simulink model "full_modek"  (R2024b)
settings: Solver=VariableStepAuto  StartTime=0.0  StopTime=20  RelTol=1e-3
values from neighbouring files (symbols this model uses):
  C = [1 0 0 0; 0 1 0 0]    [Car_test_UDP.m]    (also in Final_Code_GPS.m; Final_Code_plotting_reset_kalman.m; KalmanFilter.m)
undefined symbols (not defined in the file or in its folder): Sim3dSensor
libraries: sim3dautolib x4, sim3dcameralib x1, sim3dlib x1
settings Model: Creator=The MathWorks, Inc.  LastModifiedBy=ritvi
settings SolverCC: AlgebraicLoopSolver=TrustRegion
settings OptimizationCC: ReuseModelBlockBuffer=off
settings DebuggingCC: UnconnectedInputMsg=warning  UnconnectedOutputMsg=warning  UnconnectedLineMsg=warning  SymbolicDimsDataTypeCodeGenerationDiagnostic=none
settings ModelReferenceCC: EnableRefExpFcnMdlSchedulingChecks=on
settings RTWCC: GPUComputeCapability=3.5  DLArmComputeVersion=19.05

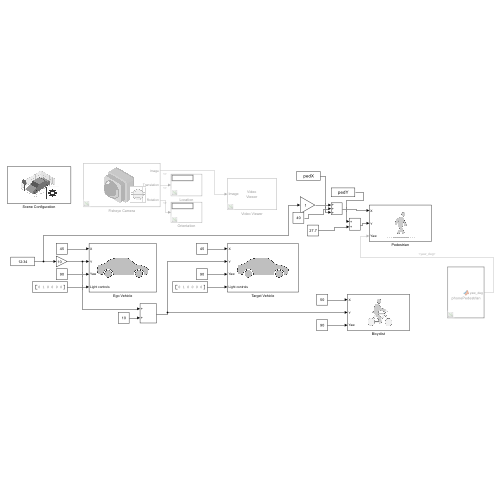
[thumbnail: Simulink's stored preview of the top-level diagram]
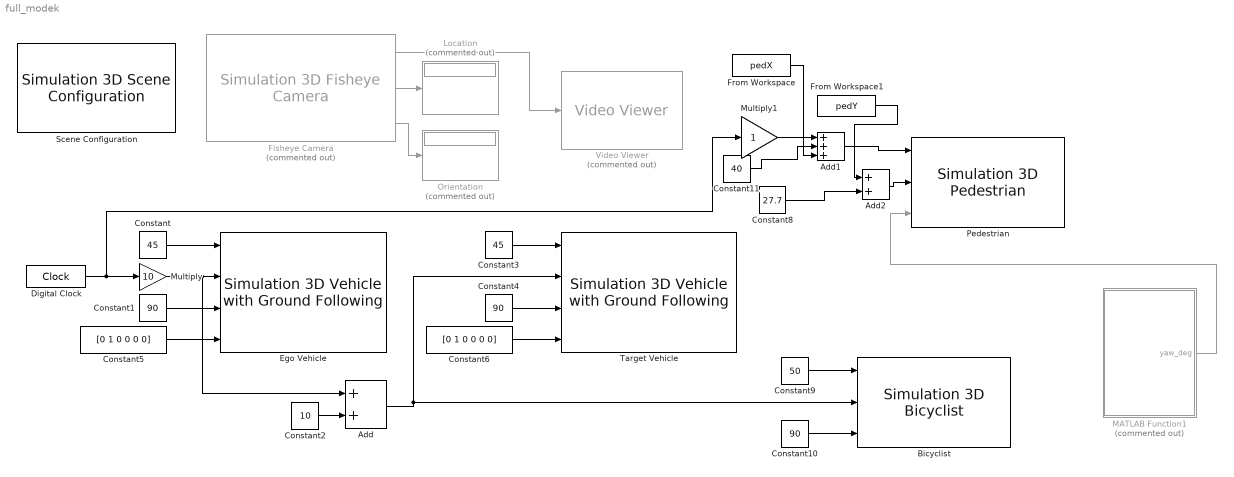
== system full_modek ==
  Add : Sum
  Add1 : Sum  Inputs=+++
  Add2 : Sum
  Bicyclist : sim3dautolib/Simulation 3D Bicyclist  Priority=-1  Scale=[1, 1, 1]  InitialPos=[0, 0, 0]  InitialRot=[0, 0, 0]  ActorName=SimulinkBicyclist1  SampleTime=-1  ActorType=SimulinkBicyclist  ActorTag=SimulinkBicyclist1  ID=1  aMode=3  CoordinateScheme=ISO  TransformOutportEnabled=off
      settings: LibrarySourceBlock=drivingsim3d/Simulation 3D Bicyclist
  Constant : Constant  Value=45
  Constant1 : Constant  Value=90
  Constant10 : Constant  Value=90
  Constant11 : Constant  Value=40
  Constant2 : Constant  Value=10
  Constant3 : Constant  Value=45
  Constant4 : Constant  Value=90
  Constant5 : Constant  Value=[0 1 0 0 0 0]
  Constant6 : Constant  Value=[0 1 0 0 0 0]
  Constant8 : Constant  Value=27.7
  Constant9 : Constant  Value=50
  Digital Clock : DigitalClock  SampleTime=0.01
  Ego Vehicle : sim3dautolib/Simulation 3D Vehicle with Ground Following  Priority=-1  PassVehMesh=Hatchback  MeshPath=/MathWorksSimulation/Vehicles/Muscle/Meshes/SK_MuscleCar.SK_MuscleCar  TrackWidth=1.9  WheelBase=3  WheelRadius=0.35  VehColor=Red  InitialPos=[45, 0, 0]  InitialRot=[0, 0, 90]  ActorName=EgoVehicle  SampleTime=-1  ActorType=SimulinkVehicle  ID=C  aMode=3  ActorTag=EgoVehicle  CoordinateScheme=ISO  VehLightsControl=on  HeadlightColor=[ 1, 1, 1 ]  HighBeamIntensity=100000  LowBeamIntensity=60000  HighBeamConeAngle=70  LowBeamConeAngle=70  LeftHeadlightOrientation=[ 0, 0 ]  RightHeadlightOrientation=[ 0, 0 ]  BrakelightIntensity=500  ReverselightIntensity=500  SignallightIntensity=500  SignallightPeriod=1  SignalPulseWidth=50  TransformOutportEnabled=off
      settings: LibrarySourceBlock=drivingsim3d/Simulation 3D Vehicle with Ground Following
  Fisheye Camera : sim3dcameralib/Simulation 3D Fisheye Camera  Priority=1  Commented=on  sensorTag=Sim3dSensor�  sensorId=1  sensorName=Sim3dSensor�  vehTagList={'EgoVehicle';'Scene Origin';'TargetVehicle'}  vehTag=EgoVehicle  mountLoc=Roof center  offsetFlag=off  tmountOffset=[0, 0, 0]  extTmount=off  rmountOffset=[0, 0, 0]  extRmount=off  OpticalCenter=[640, 360]  ImageSize=[720, 1280]  RadialDistortion=[320, -0.0005, 0, 0]  StretchMatrix=[1, 0; 0, 1]  TransformOutportEnabled=on  SampleTime=-1  mountPoint=[0 0 1.56]  mountOrientation=[0 0 0]  aMode=3  ID=1
      settings: LibrarySourceBlock=drivingsim3d/Simulation 3D Fisheye Camera
  From Workspace : FromWorkspace  VariableName=pedX
  From Workspace1 : FromWorkspace  VariableName=pedY
  Location : Display  Commented=on
  MATLAB Function1 : MATLAB Function  Commented=on  TreatAsAtomicUnit=on
  Multiply : Gain  Gain=10
  Multiply1 : Gain
  Orientation : Display  Commented=on
  Pedestrian : sim3dautolib/Simulation 3D Pedestrian  Priority=-1  PedestrianType=Female 1  Scale=[1, 1, 1]  InitialPos=[0, 0, 0]  InitialYaw=0  ActorName=SimulinkPedestrian1  SampleTime=-1  ActorType=SimulinkPedestrian  ActorTag=SimulinkPedestrian1  ID=1  aMode=3  CoordinateScheme=ISO  TransformOutportEnabled=off
      settings: LibrarySourceBlock=drivingsim3d/Simulation 3D Pedestrian
  Scene Configuration : sim3dlib/Simulation 3D Scene Configuration  Priority=0  ProjectFormat=Unreal Editor  SceneDesc=Large parking lot  ProjectName=C:\Program Files\MATLAB\R2024b\toolbox\shared\sim3d_projects\automotive_project_windows\UE\WindowsNoEditor\VehicleSimulation.exe  ScenePath=/Game/Maps/HwStrght  UEProjPath=C:\Local\AutoVrtlEnv\AutoVrtlEnv.uproject  EnableOpenDRIVE=off  vehTagList={'Custom';'EgoVehicle';'Scene Origin';'TargetVehicle'}  vehTag=EgoVehicle  FreeCameraInitialTranslation=[0, 0, 0]  FreeCameraDefaultInitialTranslation=[-6, 0, 2]  FreeCameraInitialRotation=[0, 0, 0]  FreeCameraDefaultInitialRotation=[0, -15, 0]  OpVisEn=off  Ts=1/60  EnableWindow=on  EnableRemoteAccess=off  EnableWeather=off  SunAzimuth=183.600  SunAltitude=0.0  EnableGeospatialSun=off  Latitude=0  Longitude=0  Date=2023-01-01  Time=10:30:00  GeoTimeZone=-5.0  SunDaylightSaving=off  wind=1  clouds=50.0  EnableVolumetricClouds=off  CloudCoverage=0  CloudAltitude=6  fog=0.0  rain=18.0  RaindropsEffect=off  SnowDensity=0  EnableGeospatial=off  UseTrueOrigin=off  OriginHeight=200  OriginLatitude=40.744652  OriginLongitude=-73.988864  MapStyle=Aerial  AdditionalAssetIDs=[]  UseAdvancedSunSky=off  SolarTime=11  TimeZone=-5  Day=21  Month=9  Year=2022  UseDaylightSavingTime=on  DSTStartDay=10  DSTStartMonth=3  DSTEndDay=3  DSTEndMonth=11  DSTSwitchHour=2  sensorTag=MainCamera2  sensorId=2  sensorName=MainCamera2  mountLoc=Origin  offsetFlag=off  tmountOffset=[0, 0, 0]  rmountOffset=[0, 0, 0]  HorizontalResolution=1280  VerticalResolution=720  HorizontalFOV=60  mountPoint=[0 0 0]  mountOrientation=[0 0 0]  aMode=3  ID=2  GeoTrigger=Inactive
      settings: LibrarySourceBlock=drivingsim3d/Simulation 3D Scene Configuration
  Target Vehicle : sim3dautolib/Simulation 3D Vehicle with Ground Following  Priority=-1  PassVehMesh=Sport utility vehicle  MeshPath=/MathWorksSimulation/Vehicles/Muscle/Meshes/SK_MuscleCar.SK_MuscleCar  TrackWidth=1.9  WheelBase=3  WheelRadius=0.35  VehColor=Green  InitialPos=[45, 10, 0]  InitialRot=[0, 0, 90]  ActorName=TargetVehicle  SampleTime=-1  ActorType=SimulinkVehicle  ID=C  aMode=3  ActorTag=TargetVehicle  CoordinateScheme=ISO  VehLightsControl=on  HeadlightColor=[ 1, 1, 1 ]  HighBeamIntensity=100000  LowBeamIntensity=60000  HighBeamConeAngle=70  LowBeamConeAngle=70  LeftHeadlightOrientation=[ 0, 0 ]  RightHeadlightOrientation=[ 0, 0 ]  BrakelightIntensity=500  ReverselightIntensity=500  SignallightIntensity=500  SignallightPeriod=1  SignalPulseWidth=50  TransformOutportEnabled=off
      settings: LibrarySourceBlock=drivingsim3d/Simulation 3D Vehicle with Ground Following
  Video Viewer : VideoViewer  Commented=on  FigPos=[993.8 1062.8 530.4 429.6]
  wires:
  Multiply/1 -> Add/1, Ego Vehicle/2
  Constant/1 -> Ego Vehicle/1
  Constant1/1 -> Ego Vehicle/3
  Constant2/1 -> Add/2
  Add/1 -> Target Vehicle/2, Bicyclist/2
  Fisheye Camera/1 -> Video Viewer/1
  Digital Clock/1 -> Multiply1/1, Multiply/1
  Fisheye Camera/2 -> Location/1
  Fisheye Camera/3 -> Orientation/1
  Constant3/1 -> Target Vehicle/1
  Constant4/1 -> Target Vehicle/3
  Constant5/1 -> Ego Vehicle/4
  Constant6/1 -> Target Vehicle/4
  MATLAB Function1/1(yaw_deg) -> Pedestrian/3
  Constant9/1 -> Bicyclist/1
  Constant10/1 -> Bicyclist/3
  Multiply1/1 -> Add1/1
  Add1/1 -> Pedestrian/1
  Constant11/1 -> Add1/2
  From Workspace/1 -> Add1/3
  Add2/1 -> Pedestrian/2
  Constant8/1 -> Add2/2
  From Workspace1/1 -> Add2/1

== matlab function full_modek/MATLAB Function1 ==
  data: yaw_deg output
function yaw_deg  = phonePedestrian
%#codegen

% Read MATLAB workspace value
coder.extrinsic('evalin');

% -------------------------------------------------
% PARAMETERS (tune if needed)
% -------------------------------------------------
v  = 1.2;        % walking speed (m/s)
Ts = 0.02;       % simulation step (s)

% -------------------------------------------------
% STATE (persistent)
% -------------------------------------------------
persistent yaw x_pos y_pos
if isempty(yaw)
    yaw   = 0.0;   % radians
    x_pos = 0.0;   % meters
    y_pos = 0.0;   % meters
end

% -------------------------------------------------
% INPUT: phone gyro (rad/s)
% -------------------------------------------------
wz = 0.0;
wz = evalin('base','YawRate');

% -------------------------------------------------
% UPDATE STATE
% -------------------------------------------------
yaw = yaw + wz * Ts;

x_pos = x_pos + v * cos(yaw) * Ts;
y_pos = y_pos + v * sin(yaw) * Ts;

% -------------------------------------------------
% OUTPUTS
% -------------------------------------------------
x = x_pos;
y = y_pos;
yaw_deg = yaw * 180/pi;   % Pedestrian expects degrees
